simulink model "test_diff"  (R2023b)
settings: Solver=VariableStepAuto  StartTime=0.0  StopTime=10.0  RelTol=1e-3
libraries: audiosources x2, matrix_library x2, dspsnks4 x1
settings Model: Creator=Thinkpad  LastModifiedBy=Thinkpad

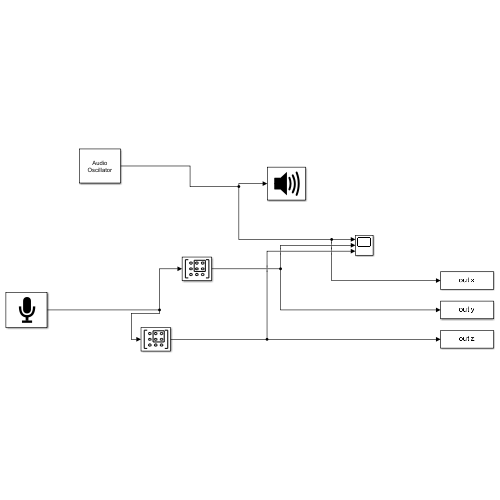
[thumbnail: Simulink's stored preview of the top-level diagram]
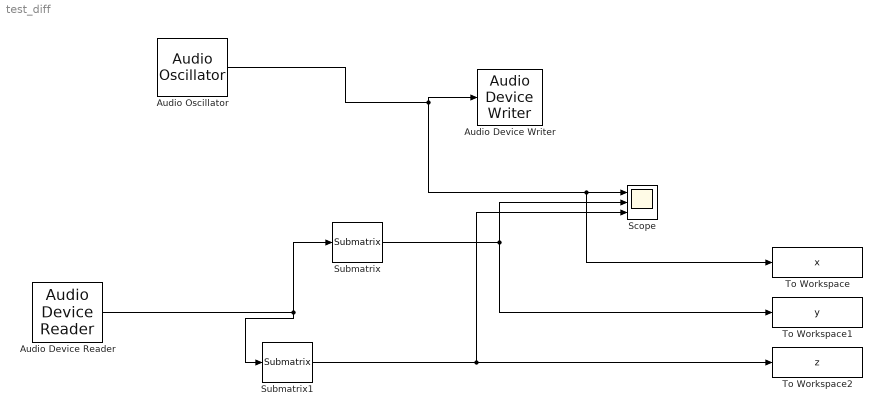
== system test_diff ==
  Audio Device Reader : audiosources/Audio Device Reader  Driver=DirectSound  Device=Default  SampleRate=48000  NumChannels=2  SamplesPerFrame=1024  BitDepth=16-bit integer  NumBuffers=10  DefaultInputChannelMapping=on  InputChannelMapping=1:2  OutputNumOverrunSamples=off  OutputDataType=double  DriverIdx=1  DeviceWarnFlag=麦克风 (Scarlett 2i2 USB)
  Audio Device Writer : dspsnks4/Audio Device Writer  Driver=DirectSound  Device=Default  InheritSampleRate=on  SampleRate=44100  BitDepth=16-bit integer  BufferSize=4096  NumBuffers=10  DefaultOutputChannelMapping=on  OutputChannelMapping=1:2  OutputNumUnderrunSamples=off  DriverIdx=1  DeviceWarnFlag=扬声器 (Scarlett 2i2 USB)
  Audio Oscillator : audiosources/Audio Oscillator  FrequencyPort=off  Frequency=100  AmplitudePort=off  Amplitude=1  DCOffsetPort=off  PhaseOffset=0  DCOffset=0  WidthPort=off  Width=1  DutyCyclePort=off  DutyCycle=0.5  SampsPerFrame=1024  Fs=48000  OutputDataType=double  SimulateUsing=Code generation
      settings: SignalType=sine
  Scope : Scope  NumInputPorts=3
  Submatrix : matrix_library/Submatrix  RowSpan=All rows  RowStartMode=First  RowStartIndex=1  RowEndMode=Last  RowEndIndex=1  ColSpan=One column  ColStartMode=First  ColStartIndex=1  ColEndMode=Last  ColEndIndex=1
  Submatrix1 : matrix_library/Submatrix  RowSpan=All rows  RowStartMode=First  RowStartIndex=1  RowEndMode=Last  RowEndIndex=1  ColSpan=One column  ColStartMode=Last  ColStartIndex=1  ColEndMode=Last  ColEndIndex=1
  To Workspace : ToWorkspace  VariableName=x  SampleTime=-1
      settings: Save2DSignal=2-D array (concatenate along first dimension)
  To Workspace1 : ToWorkspace  VariableName=y  SampleTime=-1
      settings: Save2DSignal=2-D array (concatenate along first dimension)
  To Workspace2 : ToWorkspace  VariableName=z  SampleTime=-1
      settings: Save2DSignal=2-D array (concatenate along first dimension)
  wires:
  Audio Device Reader/1 -> Submatrix/1, Submatrix1/1
  Submatrix/1 -> Scope/2, To Workspace1/1
  Audio Oscillator/1 -> Audio Device Writer/1, To Workspace/1, Scope/1
  Submatrix1/1 -> Scope/3, To Workspace2/1
